simulink library "qss_tb_library_aalto"  (Simulink 8.3)
settings: Solver=ode45  SolverMode=SingleTasking  StartTime=0.0  StopTime=1220  RelTol=1e-3
undefined symbols (not defined in the file): c_BT_E1, c_BT_E2, c_BT_E3, c_BT_E4, c_BT_L1, c_BT_L2, c_BT_L3, c_BT_L4, cap_BT, cc_done, delta_h_C_air, DiscIntNeverNeededParam, dw_GG_c, eff_FC_max, eta_EG_map, eta_EM_map, g, h, H_o_m, H_u, I_BT_max, i_FC_in, i_FC_max, k1, k2, k3, k4, k_cs, M_air, manual_gearbox, P_CVT_opt, power_max, Q_BT_0, Q_BT_IC, Q_BT_min, Q_SC_IC, r_wheel, rchg_map_BT, rdis_map_BT, rho, rho_f, soc_map_BT, t_c, T_CE_max, T_EG_c, T_EG_max, T_EM_max, T_z, U_BT_0, V, V_CE_map, V_FC_out, voc_map_BT, w_CE_max, w_CE_upper, w_CVT_opt, w_EG_row, w_EG_upper, w_EM_row, w_EM_upper ... (+1)
libraries: simulink x4
(part 4 of 4)

== system qss_tb_library_aalto/Vehicle/Vehicle/Rolling resistance ==
  v : Inport
  Rolling resistance : Constant  Value=m_f*g*mu
  Switch : Switch  Criteria=u2 > Threshold  Threshold=eps
  To Workspace2 : ToWorkspace  VariableName=F_roll  SampleTime=-1
  standstill : Constant  Value=0
  F_roll : Outport
  wires:
  Switch/1 -> To Workspace2/1, F_roll/1
  v/1 -> Switch/2
  standstill/1 -> Switch/3
  Rolling resistance/1 -> Switch/1

== system qss_tb_library_aalto/Vehicle/Vehicle v2/Aerodynamic resistance ==
  v : Inport
  Aerodynamic resistance : Fcn  Expr=0.5*rho*cw*A_f*u^2
  To Workspace10 : ToWorkspace  VariableName=F_aero  SampleTime=-1
  F_aero : Outport  InitialOutput=0
  wires:
  Aerodynamic resistance/1 -> To Workspace10/1, F_aero/1
  v/1 -> Aerodynamic resistance/1

== system qss_tb_library_aalto/Vehicle/Vehicle v2/Average speed ==
  v : Inport
  Gain5 : Gain  Gain=0.5  SaturateOnIntegerOverflow=on  OutDataTypeStr=Inherit: Same as input  ParamDataTypeStr=Inherit: Same as input
  Sum2 : Sum  SaturateOnIntegerOverflow=on  InputSameDT=on  OutDataTypeStr=Inherit: Same as first input
  Unit Delay : UnitDelay  SampleTime=h
  v_a : Outport  InitialOutput=0
  wires:
  v/1 -> Unit Delay/1, Sum2/1
  Gain5/1 -> v_a/1
  Sum2/1 -> Gain5/1
  Unit Delay/1 -> Sum2/2

== system qss_tb_library_aalto/Vehicle/Vehicle v2/Inertia ==
  d_v : Inport
  Inertia : Fcn  Expr=m_f*(1+mt2m_f)*u/h
  To Workspace10 : ToWorkspace  VariableName=F_iner  SampleTime=-1
  F_iner : Outport  InitialOutput=0
  wires:
  d_v/1 -> Inertia/1
  Inertia/1 -> To Workspace10/1, F_iner/1

== system qss_tb_library_aalto/Vehicle/Vehicle v2/Rolling resistance ==
  v : Inport
  Rolling resistance : Constant  Value=m_f*g*mu
  Switch : Switch  Criteria=u2 > Threshold  Threshold=eps
  To Workspace2 : ToWorkspace  VariableName=F_roll  SampleTime=-1
  standstill : Constant  Value=0
  F_roll : Outport
  wires:
  Rolling resistance/1 -> Switch/1
  standstill/1 -> Switch/3
  v/1 -> Switch/2
  Switch/1 -> F_roll/1, To Workspace2/1

== system qss_tb_library_aalto/Controller/Battery Controller/Geno-Group On/Clock ==
  Constant : Constant
  Sum : Sum  Inputs=+-  SaturateOnIntegerOverflow=on  InputSameDT=on  OutDataTypeStr=Inherit: Same as first input
  Unit Delay : UnitDelay  SampleTime=duration
  out_1 : Outport  InitialOutput=0
  wires:
  Constant/1 -> Sum/1
  Sum/1 -> Unit Delay/1, out_1/1
  Unit Delay/1 -> Sum/2

== system qss_tb_library_aalto/Controller/Gen-set Controller v2/Engine start control/Engine on off ==
  S : Inport
  R : Inport  Port=2
  Demux : Demux  Outputs=2
  Logic : CombinatorialLogic  TruthTable=[0 1;0 1;1 0;0 1;1 0;0 1;1 0;1 0]
  Memory : Memory  InheritSampleTime=on
  Mux : Mux  Inputs=3
  Q : Outport  InitialOutput=0
  !Q : Outport  Port=2  InitialOutput=1
  wires:
  Mux/1 -> Logic/1
  Logic/1 -> Demux/1
  Demux/2 -> !Q/1
  Demux/1 -> Q/1, Memory/1
  Memory/1 -> Mux/1
  S/1 -> Mux/2
  R/1 -> Mux/3

== system qss_tb_library_aalto/Controller/Gen-set Controller v2/Engine start control/tempo ==
  flag : Inport
  time : Inport  Port=2
  S-R Flip-Flop : Subsystem  mask(SRFlipFlop){initial_condition=1}
      mask prompts: initial_condition "Initial condition (state of Q):"
      mask help: S-R Flip-Flop Block
      mask Help: web([docroot '/toolbox/simulink/ref_extras/srflipflop.html'])
  Terminator : Terminator
  Unit Delay : UnitDelay  SampleTime=h
  __Logical Operator2 : Logic
  __Logical Operator3 : Logic  Operator=NOT
  __Terminator : Terminator
  counter : DiscreteIntegrator  ExternalReset=rising  SampleTime=h  ICPrevOutput=DiscIntNeverNeededParam  ICPrevScaledInput=DiscIntNeverNeededParam
  end of tempo : RelationalOperator  InputSameDT=on
  tempo ok --> 1 : Subsystem  mask(SRFlipFlop){initial_condition=0, Tech=h}
      mask prompts: initial_condition "Initial condition:"; Tech "pas d'echantillonage"
      mask help: S-R Flip Flop Block
  tempo : Outport
  wires:
  S-R Flip-Flop/1(Q) -> counter/1
  flag/1 -> __Logical Operator2/1, tempo ok --> 1/1(S)
  S-R Flip-Flop/2(!Q) -> __Terminator/1
  __Logical Operator2/1 -> S-R Flip-Flop/1(S)
  __Logical Operator3/1 -> __Logical Operator2/2
  time/1 -> end of tempo/2
  end of tempo/1 -> Unit Delay/1, tempo ok --> 1/2(R)
  Unit Delay/1 -> __Logical Operator3/1, S-R Flip-Flop/2(R), counter/2
  counter/1 -> end of tempo/1
  tempo ok --> 1/2(!Q) -> Terminator/1
  tempo ok --> 1/1(Q) -> tempo/1

== system qss_tb_library_aalto/Controller/Gen-set Controller/Engine start control/Engine on off ==
  S : Inport
  R : Inport  Port=2
  Demux : Demux  Outputs=2
  Logic : CombinatorialLogic  TruthTable=[0 1;0 1;1 0;0 1;1 0;0 1;1 0;1 0]
  Memory : Memory  InheritSampleTime=on
  Mux : Mux  Inputs=3
  Q : Outport  InitialOutput=0
  !Q : Outport  Port=2  InitialOutput=1
  wires:
  R/1 -> Mux/3
  S/1 -> Mux/2
  Memory/1 -> Mux/1
  Demux/1 -> Memory/1, Q/1
  Demux/2 -> !Q/1
  Logic/1 -> Demux/1
  Mux/1 -> Logic/1

== system qss_tb_library_aalto/Controller/Gen-set Controller/Engine start control/tempo ==
  flag : Inport
  time : Inport  Port=2
  S-R Flip-Flop : Subsystem  mask(SRFlipFlop){initial_condition=1}
      mask prompts: initial_condition "Initial condition (state of Q):"
      mask help: S-R Flip-Flop Block
      mask Help: web([docroot '/toolbox/simulink/ref_extras/srflipflop.html'])
  Terminator : Terminator
  Unit Delay : UnitDelay  SampleTime=h
  __Logical Operator2 : Logic
  __Logical Operator3 : Logic  Operator=NOT
  __Terminator : Terminator
  counter : DiscreteIntegrator  ExternalReset=rising  SampleTime=h  ICPrevOutput=DiscIntNeverNeededParam  ICPrevScaledInput=DiscIntNeverNeededParam
  end of tempo : RelationalOperator  InputSameDT=on
  tempo ok --> 1 : Subsystem  mask(SRFlipFlop){initial_condition=0, Tech=h}
      mask prompts: initial_condition "Initial condition:"; Tech "pas d'echantillonage"
      mask help: S-R Flip Flop Block
  tempo : Outport
  wires:
  tempo ok --> 1/1(Q) -> tempo/1
  tempo ok --> 1/2(!Q) -> Terminator/1
  counter/1 -> end of tempo/1
  Unit Delay/1 -> counter/2, S-R Flip-Flop/2(R), __Logical Operator3/1
  end of tempo/1 -> tempo ok --> 1/2(R), Unit Delay/1
  time/1 -> end of tempo/2
  __Logical Operator3/1 -> __Logical Operator2/2
  __Logical Operator2/1 -> S-R Flip-Flop/1(S)
  S-R Flip-Flop/2(!Q) -> __Terminator/1
  flag/1 -> tempo ok --> 1/1(S), __Logical Operator2/1
  S-R Flip-Flop/1(Q) -> counter/1

== system qss_tb_library_aalto/Energy Buffer/Battery/Battery voltage/Charging ==
  Q_BT : Inport
  P_BT : Inport  Port=2
  Enable : EnablePort
  Constant4 : Constant  Value=Q_BT_0
  Fcn : Fcn  Expr=(c_BT_L3*u[1]+c_BT_L1+sqrt((c_BT_L3*u[1]+c_BT_L1)^2+4*(c_BT_L4*u[1]+c_BT_L2)*(-u[2])))/2
  Gain2 : Gain  Gain=1/Q_BT_0  SaturateOnIntegerOverflow=on  OutDataTypeStr=Inherit: Same as input  ParamDataTypeStr=Inherit: Same as input
  Gain4 : Gain  Gain=1/I_0  SaturateOnIntegerOverflow=on  OutDataTypeStr=Inherit: Same as input  ParamDataTypeStr=Inherit: Same as input
  Mux : Mux  Inputs=2
  Sum4 : Sum  Inputs=-+  SaturateOnIntegerOverflow=on  InputSameDT=on  OutDataTypeStr=Inherit: Same as first input
  U_BT_L : Outport  InitialOutput=0
  wires:
  Gain4/1 -> Mux/2
  Gain2/1 -> Mux/1
  Sum4/1 -> Gain2/1
  Q_BT/1 -> Sum4/1
  Constant4/1 -> Sum4/2
  P_BT/1 -> Gain4/1
  Mux/1 -> Fcn/1
  Fcn/1 -> U_BT_L/1

== system qss_tb_library_aalto/Energy Buffer/Battery/Battery voltage/Discharging ==
  note: q
  note: P/I_0
  Q_BT : Inport
  P_BT : Inport  Port=2
  Enable : EnablePort
  Constant6 : Constant  Value=Q_BT_0
  Fcn : Fcn  Expr=(c_BT_E3*u[1]+c_BT_E1+sqrt((c_BT_E3*u[1]+c_BT_E1)^2+4*(c_BT_E4*u[1]+c_BT_E2)*(-u[2])))/2
  Gain4 : Gain  Gain=1/Q_BT_0  SaturateOnIntegerOverflow=on  OutDataTypeStr=Inherit: Same as input  ParamDataTypeStr=Inherit: Same as input
  Gain5 : Gain  Gain=1/I_0  SaturateOnIntegerOverflow=on  OutDataTypeStr=Inherit: Same as input  ParamDataTypeStr=Inherit: Same as input
  Mux : Mux  Inputs=2
  Sum7 : Sum  Inputs=-+  SaturateOnIntegerOverflow=on  InputSameDT=on  OutDataTypeStr=Inherit: Same as first input
  U_BT_E : Outport  InitialOutput=0
  wires:
  Fcn/1 -> U_BT_E/1
  Sum7/1 -> Gain4/1
  Q_BT/1 -> Sum7/1
  Constant6/1 -> Sum7/2
  P_BT/1 -> Gain5/1
  Gain4/1 -> Mux/1
  Gain5/1 -> Mux/2
  Mux/1 -> Fcn/1

== system qss_tb_library_aalto/Energy Buffer/Battery/Battery voltage/Enable charging ==
  P_BT : Inport
  Gain : Gain  Gain=-1  SaturateOnIntegerOverflow=on  OutDataTypeStr=Inherit: Same as input  ParamDataTypeStr=Inherit: Same as input
  Saturation : Saturate  UpperLimit=0  LowerLimit=-inf
  Sign : Signum
  e_E : Outport  InitialOutput=0
  wires:
  P_BT/1 -> Saturation/1
  Sign/1 -> e_E/1
  Saturation/1 -> Gain/1
  Gain/1 -> Sign/1

== system qss_tb_library_aalto/Energy Buffer/Battery/Battery voltage/Enable discharging ==
  P_BT : Inport
  Saturation : Saturate  UpperLimit=inf  LowerLimit=0
  Sign : Signum
  e_E : Outport  InitialOutput=0
  wires:
  P_BT/1 -> Saturation/1
  Sign/1 -> e_E/1
  Saturation/1 -> Sign/1

== system qss_tb_library_aalto/Energy Buffer/Battery/Battery voltage/Enable idle ==
  P_BT : Inport
  Abs : Abs  SaturateOnIntegerOverflow=on
  Constant : Constant
  Sign : Signum
  Sum4 : Sum  Inputs=-+  SaturateOnIntegerOverflow=on  InputSameDT=on  OutDataTypeStr=Inherit: Same as first input
  e_Z : Outport  InitialOutput=0
  wires:
  P_BT/1 -> Sign/1
  Sign/1 -> Abs/1
  Abs/1 -> Sum4/1
  Sum4/1 -> e_Z/1
  Constant/1 -> Sum4/2

== system qss_tb_library_aalto/Energy Buffer/Battery/Battery voltage/Idle ==
  Q_BT : Inport
  Enable : EnablePort  StatesWhenEnabling=reset
  Constant : Constant  Value=c_BT_L1
  Constant6 : Constant  Value=Q_BT_0
  Gain4 : Gain  Gain=c_BT_L3/Q_BT_0  SaturateOnIntegerOverflow=on  OutDataTypeStr=Inherit: Same as input  ParamDataTypeStr=Inherit: Same as input
  Sum7 : Sum  Inputs=-+  SaturateOnIntegerOverflow=on  InputSameDT=on  OutDataTypeStr=Inherit: Same as first input
  Sum8 : Sum  SaturateOnIntegerOverflow=on  InputSameDT=on  OutDataTypeStr=Inherit: Same as first input
  U_BT_E : Outport  InitialOutput=0
  wires:
  Sum7/1 -> Gain4/1
  Q_BT/1 -> Sum7/1
  Constant6/1 -> Sum7/2
  Gain4/1 -> Sum8/1
  Constant/1 -> Sum8/2
  Sum8/1 -> U_BT_E/1

== system qss_tb_library_aalto/Energy Buffer/Battery/Battery voltage/Supervision battery ==
  Q_BT : Inport
  U_BT : Inport  Port=2
  I_BT : Inport  Port=3
  Abs : Abs  SaturateOnIntegerOverflow=on
  Constant4 : Constant  Value=Q_BT_0
  Constant6 : Constant  Value=c_BT_E1
  Constant7 : Constant  Value=I_BT_max
  Gain2 : Gain  Gain=c_BT_E3/Q_BT_0  SaturateOnIntegerOverflow=on  OutDataTypeStr=Inherit: Same as input  ParamDataTypeStr=Inherit: Same as input
  Gain3 : Gain  Gain=2  SaturateOnIntegerOverflow=on  OutDataTypeStr=Inherit: Same as input  ParamDataTypeStr=Inherit: Same as input
  Saturation : Saturate  UpperLimit=0  LowerLimit=-inf
  Saturation1 : Saturate  UpperLimit=0  LowerLimit=-inf
  Stop Simulation : Stop
  Stop Simulation1 : Stop
  Sum1 : Sum  Inputs=-+  SaturateOnIntegerOverflow=on  InputSameDT=on  OutDataTypeStr=Inherit: Same as first input
  Sum2 : Sum  Inputs=+-  SaturateOnIntegerOverflow=on  InputSameDT=on  OutDataTypeStr=Inherit: Same as first input
  Sum3 : Sum  SaturateOnIntegerOverflow=on  InputSameDT=on  OutDataTypeStr=Inherit: Same as first input
  Sum4 : Sum  Inputs=-+  SaturateOnIntegerOverflow=on  InputSameDT=on  OutDataTypeStr=Inherit: Same as first input
  wires:
  Sum3/1 -> Sum1/1
  U_BT/1 -> Gain3/1
  Gain3/1 -> Sum1/2
  Saturation/1 -> Stop Simulation1/1
  Saturation1/1 -> Stop Simulation/1
  Sum1/1 -> Saturation1/1
  Constant6/1 -> Sum3/2
  Gain2/1 -> Sum3/1
  Sum4/1 -> Gain2/1
  Q_BT/1 -> Sum4/1
  Constant4/1 -> Sum4/2
  Constant7/1 -> Sum2/1
  Sum2/1 -> Saturation/1
  I_BT/1 -> Abs/1
  Abs/1 -> Sum2/2

== system qss_tb_library_aalto/Energy Buffer/Battery v2/cell model/soc calculation ==
  current : Inport
  (sec->hrs) : Gain  Gain=1/3600  SaturateOnIntegerOverflow=on  OutDataTypeStr=Inherit: Same as input  ParamDataTypeStr=Inherit: Same as input
  (sec->hrs)1 : Gain  Gain=-1  SaturateOnIntegerOverflow=on  OutDataTypeStr=Inherit: Same as input  ParamDataTypeStr=Inherit: Same as input
  0 <= SOC <= 1 : Saturate  UpperLimit=1  LowerLimit=0
  Constant : Constant  Value=init_soc_BT
  Constant1 : Constant  Value=cap_BT
  Discrete-Time Integrator : DiscreteIntegrator  InitialConditionSource=external  ICPrevOutput=DiscIntNeverNeededParam  ICPrevScaledInput=DiscIntNeverNeededParam
  Divide : Product  Inputs=*/  RndMeth=Zero
  Product : Product  RndMeth=Zero
  soc : Outport
  wires:
  current/1 -> (sec->hrs)/1
  0 <= SOC <= 1/1 -> soc/1
  (sec->hrs)/1 -> (sec->hrs)1/1
  Discrete-Time Integrator/1 -> Divide/1
  Divide/1 -> 0 <= SOC <= 1/1
  Constant/1 -> Product/1
  Product/1 -> Discrete-Time Integrator/2
  (sec->hrs)1/1 -> Discrete-Time Integrator/1
  Constant1/1 -> Product/2, Divide/2

== system qss_tb_library_aalto/Energy Buffer/Battery v2/cell model/voltage calculation ==
  note: Volt = Voc - Rint*I
  SOC (prev) : Inport
  Current : Inport  Port=2
  Product2 : Product  SaturateOnIntegerOverflow=on  InputSameDT=on  OutDataTypeStr=Inherit: Same as first input
  Rchg : Lookup  InputValues=soc_map_BT  Table=rchg_map_BT  SaturateOnIntegerOverflow=on
  Rdis : Lookup  InputValues=soc_map_BT  Table=rdis_map_BT  SaturateOnIntegerOverflow=on
  Sum1 : Sum  Inputs=+-  SaturateOnIntegerOverflow=on  InputSameDT=on  OutDataTypeStr=Inherit: Same as first input
  Switch : Switch  SaturateOnIntegerOverflow=on  InputSameDT=on
  Switch1 : Switch  SaturateOnIntegerOverflow=on  InputSameDT=on
  VOC : Lookup  InputValues=soc_map_BT  Table=voc_map_BT  SaturateOnIntegerOverflow=on
  coulombic efficiency : Gain  Gain=0.99
  Voc : Outport  InitialOutput=0
  voltage : Outport  Port=2  InitialOutput=0
  Rint : Outport  Port=3  InitialOutput=0
  wires:
  Switch/1 -> Rint/1, Product2/2
  Rdis/1 -> Switch/1
  Rchg/1 -> Switch/3
  VOC/1 -> Voc/1, Sum1/1
  SOC (prev)/1 -> VOC/1, Rdis/1, Rchg/1
  Product2/1 -> Sum1/2
  Sum1/1 -> voltage/1
  Switch1/1 -> Switch/2, Product2/1
  Current/1 -> Switch1/2, Switch1/1, coulombic efficiency/1
  coulombic efficiency/1 -> Switch1/3

== system qss_tb_library_aalto/Energy Buffer/Battery v3/cell model/soc calculation ==
  current : Inport
  (sec->hrs) : Gain  Gain=1/3600  SaturateOnIntegerOverflow=on  OutDataTypeStr=Inherit: Same as input  ParamDataTypeStr=Inherit: Same as input
  (sec->hrs)1 : Gain  Gain=-1  SaturateOnIntegerOverflow=on  OutDataTypeStr=Inherit: Same as input  ParamDataTypeStr=Inherit: Same as input
  0 <= SOC <= 1 : Saturate  UpperLimit=1  LowerLimit=0
  Constant : Constant  Value=init_soc_BT
  Constant1 : Constant  Value=cap_BT
  Discrete-Time Integrator : DiscreteIntegrator  InitialConditionSource=external  ICPrevOutput=DiscIntNeverNeededParam  ICPrevScaledInput=DiscIntNeverNeededParam
  Divide : Product  Inputs=*/  RndMeth=Zero
  Product : Product  RndMeth=Zero
  soc : Outport
  wires:
  Constant1/1 -> Divide/2, Product/2
  (sec->hrs)1/1 -> Discrete-Time Integrator/1
  Product/1 -> Discrete-Time Integrator/2
  Constant/1 -> Product/1
  Divide/1 -> 0 <= SOC <= 1/1
  Discrete-Time Integrator/1 -> Divide/1
  (sec->hrs)/1 -> (sec->hrs)1/1
  0 <= SOC <= 1/1 -> soc/1
  current/1 -> (sec->hrs)/1

== system qss_tb_library_aalto/Energy Buffer/Battery v3/cell model/voltage calculation ==
  note: Volt = Voc - Rint*I
  SOC (prev) : Inport
  Current : Inport  Port=2
  Product2 : Product  SaturateOnIntegerOverflow=on  InputSameDT=on  OutDataTypeStr=Inherit: Same as first input
  Rchg : Lookup  InputValues=soc_map_BT  Table=rchg_map_BT  SaturateOnIntegerOverflow=on
  Rdis : Lookup  InputValues=soc_map_BT  Table=rdis_map_BT  SaturateOnIntegerOverflow=on
  Sum1 : Sum  Inputs=+-  SaturateOnIntegerOverflow=on  InputSameDT=on  OutDataTypeStr=Inherit: Same as first input
  Switch : Switch  SaturateOnIntegerOverflow=on  InputSameDT=on
  VOC : Lookup  InputValues=soc_map_BT  Table=voc_map_BT  SaturateOnIntegerOverflow=on
  Voc : Outport  InitialOutput=0
  voltage : Outport  Port=2  InitialOutput=0
  Rint : Outport  Port=3  InitialOutput=0
  wires:
  Current/1 -> Product2/1, Switch/2
  Sum1/1 -> voltage/1
  Product2/1 -> Sum1/2
  SOC (prev)/1 -> Rchg/1, Rdis/1, VOC/1
  VOC/1 -> Sum1/1, Voc/1
  Rchg/1 -> Switch/3
  Rdis/1 -> Switch/1
  Switch/1 -> Product2/2, Rint/1

== system qss_tb_library_aalto/Energy Converter/Combustion Engine (hybrid vehicle)/torque limit/saturation with inputs ==
  upper limit in : Inport
  signal in : Inport  Port=2
  lower limit in : Inport  Port=3
  Relational Operator : RelationalOperator  Operator=<  InputSameDT=on
  Relational Operator1 : RelationalOperator  InputSameDT=on
  Switch : Switch  Threshold=0.5  SaturateOnIntegerOverflow=on  InputSameDT=on
  Switch1 : Switch  Threshold=0.5  SaturateOnIntegerOverflow=on  InputSameDT=on
  signal out : Outport
  wires:
  Switch/1 -> Switch1/1, Relational Operator1/1
  signal in/1 -> Switch/3, Relational Operator/2
  Switch1/1 -> signal out/1
  Relational Operator1/1 -> Switch1/2
  Relational Operator/1 -> Switch/2
  lower limit in/1 -> Switch1/3, Relational Operator1/2
  upper limit in/1 -> Switch/1, Relational Operator/1

== system qss_tb_library_aalto/Energy Converter/Combustion Engine (hybrid vehicle) v2/torque limit/saturation with inputs ==
  upper limit in : Inport
  signal in : Inport  Port=2
  lower limit in : Inport  Port=3
  Relational Operator : RelationalOperator  Operator=<  InputSameDT=on
  Relational Operator1 : RelationalOperator  InputSameDT=on
  Switch : Switch  Threshold=0.5  SaturateOnIntegerOverflow=on  InputSameDT=on
  Switch1 : Switch  Threshold=0.5  SaturateOnIntegerOverflow=on  InputSameDT=on
  signal out : Outport
  wires:
  upper limit in/1 -> Relational Operator/1, Switch/1
  lower limit in/1 -> Relational Operator1/2, Switch1/3
  Relational Operator/1 -> Switch/2
  Relational Operator1/1 -> Switch1/2
  Switch1/1 -> signal out/1
  signal in/1 -> Relational Operator/2, Switch/3
  Switch/1 -> Relational Operator1/1, Switch1/1

== system qss_tb_library_aalto/Gear System/Continuously Variable Transmission/Power flow/Engine -> Wheel ==
  w_wheel : Inport
  T_wheel : Inport  Port=2
  j_CVT : Inport  Port=3
  Constant3 : Constant  Value=P_CVT0
  Constant4 : Constant  Value=inf
  Gain : Gain  Gain=e_CVT  SaturateOnIntegerOverflow=on  OutDataTypeStr=Inherit: Same as input  ParamDataTypeStr=Inherit: Same as input
  Product4 : Product  Inputs=*/  SaturateOnIntegerOverflow=on  RndMeth=Zero  InputSameDT=on  OutDataTypeStr=Inherit: Same as first input
  Product5 : Product  Inputs=/*  SaturateOnIntegerOverflow=on  RndMeth=Zero  InputSameDT=on  OutDataTypeStr=Inherit: Same as first input
  Sum1 : Sum  SaturateOnIntegerOverflow=on  InputSameDT=on  OutDataTypeStr=Inherit: Same as first input
  Switch2 : Switch  Threshold=w_wheel_min  SaturateOnIntegerOverflow=on  InputSameDT=on
  T_CVT+ : Outport  InitialOutput=0
  wires:
  Gain/1 -> Product4/2
  Product4/1 -> T_CVT+/1
  Sum1/1 -> Product4/1
  T_wheel/1 -> Sum1/2
  Product5/1 -> Sum1/1
  w_wheel/1 -> Switch2/1, Switch2/2
  Constant4/1 -> Switch2/3
  Switch2/1 -> Product5/1
  Constant3/1 -> Product5/2
  j_CVT/1 -> Gain/1

== system qss_tb_library_aalto/Gear System/Continuously Variable Transmission/Power flow/Pwer Wheel -> Engine ==
  w_wheel : Inport
  T_wheel : Inport  Port=2
  j_CVT : Inport  Port=3
  Constant1 : Constant  Value=P_CVT0
  Constant2 : Constant  Value=inf
  Gain1 : Gain  Gain=1/e_CVT  SaturateOnIntegerOverflow=on  OutDataTypeStr=Inherit: Same as input  ParamDataTypeStr=Inherit: Same as input
  Gain2 : Gain  Gain=1/e_CVT  SaturateOnIntegerOverflow=on  OutDataTypeStr=Inherit: Same as input  ParamDataTypeStr=Inherit: Same as input
  Product2 : Product  Inputs=*/  SaturateOnIntegerOverflow=on  RndMeth=Zero  InputSameDT=on  OutDataTypeStr=Inherit: Same as first input
  Product3 : Product  Inputs=/*  SaturateOnIntegerOverflow=on  RndMeth=Zero  InputSameDT=on  OutDataTypeStr=Inherit: Same as first input
  Sum : Sum  Inputs=-+  SaturateOnIntegerOverflow=on  InputSameDT=on  OutDataTypeStr=Inherit: Same as first input
  Switch1 : Switch  Threshold=w_wheel_min  SaturateOnIntegerOverflow=on  InputSameDT=on
  T_CVT- : Outport  InitialOutput=0
  wires:
  Sum/1 -> Product2/1
  Gain1/1 -> Product3/2
  Switch1/1 -> Product3/1
  T_wheel/1 -> Sum/2
  Product3/1 -> Sum/1
  Product2/1 -> T_CVT-/1
  w_wheel/1 -> Switch1/1, Switch1/2
  Constant1/1 -> Gain1/1
  Constant2/1 -> Switch1/3
  j_CVT/1 -> Gain2/1
  Gain2/1 -> Product2/2

== system qss_tb_library_aalto/Gear System/Manual Gear Box/Power flow/Engine -> Wheel ==
  w_wheel : Inport
  T_wheel : Inport  Port=2
  gear : Inport  Port=3
  Constant1 : Constant  Value=P_GT0
  Constant2 : Constant  Value=inf
  Gain : Gain  Gain=e_GT  SaturateOnIntegerOverflow=on  OutDataTypeStr=Inherit: Same as input  ParamDataTypeStr=Inherit: Same as input
  Product2 : Product  Inputs=*/  SaturateOnIntegerOverflow=on  RndMeth=Zero  InputSameDT=on  OutDataTypeStr=Inherit: Same as first input
  Product3 : Product  Inputs=/*  SaturateOnIntegerOverflow=on  RndMeth=Zero  InputSameDT=on  OutDataTypeStr=Inherit: Same as first input
  Sum : Sum  SaturateOnIntegerOverflow=on  InputSameDT=on  OutDataTypeStr=Inherit: Same as first input
  Switch1 : Switch  Threshold=w_wheel_min  SaturateOnIntegerOverflow=on  InputSameDT=on
  T_MGB+ : Outport  InitialOutput=0
  wires:
  T_wheel/1 -> Sum/2
  Product3/1 -> Sum/1
  Gain/1 -> Product2/2
  Product2/1 -> T_MGB+/1
  Sum/1 -> Product2/1
  w_wheel/1 -> Switch1/2, Switch1/1
  Constant2/1 -> Switch1/3
  Switch1/1 -> Product3/1
  Constant1/1 -> Product3/2
  gear/1 -> Gain/1

== system qss_tb_library_aalto/Gear System/Manual Gear Box/Power flow/Wheel -> Engine ==
  w_wheel : Inport
  T_wheel : Inport  Port=2
  gear : Inport  Port=3
  Constant1 : Constant  Value=P_GT0
  Constant2 : Constant  Value=inf
  Gain1 : Gain  Gain=e_GT  SaturateOnIntegerOverflow=on  OutDataTypeStr=Inherit: Same as input  ParamDataTypeStr=Inherit: Same as input
  Gain2 : Gain  Gain=1/e_GT  SaturateOnIntegerOverflow=on  OutDataTypeStr=Inherit: Same as input  ParamDataTypeStr=Inherit: Same as input
  Product2 : Product  Inputs=*/  SaturateOnIntegerOverflow=on  RndMeth=Zero  InputSameDT=on  OutDataTypeStr=Inherit: Same as first input
  Product3 : Product  Inputs=/*  SaturateOnIntegerOverflow=on  RndMeth=Zero  InputSameDT=on  OutDataTypeStr=Inherit: Same as first input
  Sum : Sum  SaturateOnIntegerOverflow=on  InputSameDT=on  OutDataTypeStr=Inherit: Same as first input
  Switch1 : Switch  Threshold=w_wheel_min  SaturateOnIntegerOverflow=on  InputSameDT=on
  T_MGB- : Outport  InitialOutput=0
  wires:
  w_wheel/1 -> Switch1/1, Switch1/2
  gear/1 -> Gain2/1
  Constant2/1 -> Switch1/3
  Switch1/1 -> Gain1/1
  Constant1/1 -> Product3/2
  T_wheel/1 -> Sum/1
  Gain2/1 -> Product2/2
  Product2/1 -> T_MGB-/1
  Product3/1 -> Sum/2
  Sum/1 -> Product2/1
  Gain1/1 -> Product3/1

== system qss_tb_library_aalto/Gear System/Simple Transmission/Power flow/Energy Engine -> Wheel ==
  w_wheel : Inport
  T_wheel : Inport  Port=2
  gear_ratio : Inport  Port=3
  Constant1 : Constant  Value=P_GT0
  Constant2 : Constant  Value=inf
  Gain : Gain  Gain=e_GT  SaturateOnIntegerOverflow=on  OutDataTypeStr=Inherit: Same as input  ParamDataTypeStr=Inherit: Same as input
  Product2 : Product  Inputs=*/  SaturateOnIntegerOverflow=on  RndMeth=Zero  InputSameDT=on  OutDataTypeStr=Inherit: Same as first input
  Product3 : Product  Inputs=/*  SaturateOnIntegerOverflow=on  RndMeth=Zero  InputSameDT=on  OutDataTypeStr=Inherit: Same as first input
  Sum : Sum  SaturateOnIntegerOverflow=on  InputSameDT=on  OutDataTypeStr=Inherit: Same as first input
  Switch1 : Switch  Threshold=w_wheel_min  SaturateOnIntegerOverflow=on  InputSameDT=on
  T_trans+ : Outport  InitialOutput=0
  wires:
  T_wheel/1 -> Sum/2
  Product3/1 -> Sum/1
  Gain/1 -> Product2/2
  Product2/1 -> T_trans+/1
  Sum/1 -> Product2/1
  w_wheel/1 -> Switch1/2, Switch1/1
  Constant2/1 -> Switch1/3
  Switch1/1 -> Product3/1
  Constant1/1 -> Product3/2
  gear_ratio/1 -> Gain/1

== system qss_tb_library_aalto/Gear System/Simple Transmission/Power flow/Energy Wheel -> Engine ==
  w_wheel : Inport
  T_wheel : Inport  Port=2
  gear_ratio : Inport  Port=3
  Constant1 : Constant  Value=P_GT0
  Constant2 : Constant  Value=inf
  Gain1 : Gain  Gain=e_GT  SaturateOnIntegerOverflow=on  OutDataTypeStr=Inherit: Same as input  ParamDataTypeStr=Inherit: Same as input
  Gain2 : Gain  Gain=1/e_GT  SaturateOnIntegerOverflow=on  OutDataTypeStr=Inherit: Same as input  ParamDataTypeStr=Inherit: Same as input
  Product2 : Product  Inputs=*/  SaturateOnIntegerOverflow=on  RndMeth=Zero  InputSameDT=on  OutDataTypeStr=Inherit: Same as first input
  Product3 : Product  Inputs=/*  SaturateOnIntegerOverflow=on  RndMeth=Zero  InputSameDT=on  OutDataTypeStr=Inherit: Same as first input
  Sum : Sum  SaturateOnIntegerOverflow=on  InputSameDT=on  OutDataTypeStr=Inherit: Same as first input
  Switch1 : Switch  Threshold=w_wheel_min  SaturateOnIntegerOverflow=on  InputSameDT=on
  T_trans- : Outport  InitialOutput=0
  wires:
  w_wheel/1 -> Switch1/1, Switch1/2
  gear_ratio/1 -> Gain2/1
  Constant2/1 -> Switch1/3
  Switch1/1 -> Gain1/1
  Constant1/1 -> Product3/2
  T_wheel/1 -> Sum/1
  Gain2/1 -> Product2/2
  Product2/1 -> T_trans-/1
  Product3/1 -> Sum/2
  Sum/1 -> Product2/1
  Gain1/1 -> Product3/1

== system qss_tb_library_aalto/Gear System/Transmission CE-EG/Power flow/Energy Engine -> Wheel ==
  w_wheel : Inport
  T_wheel : Inport  Port=2
  gear_ratio : Inport  Port=3
  Constant1 : Constant  Value=P_GT0
  Constant2 : Constant  Value=inf
  Gain1 : Gain  Gain=e_GT  SaturateOnIntegerOverflow=on  OutDataTypeStr=Inherit: Same as input  ParamDataTypeStr=Inherit: Same as input
  Lower limit : Saturate  UpperLimit=inf  LowerLimit=0
  Product2 : Product  Inputs=*/  SaturateOnIntegerOverflow=on  RndMeth=Zero  InputSameDT=on  OutDataTypeStr=Inherit: Same as first input
  Product3 : Product  Inputs=/*  SaturateOnIntegerOverflow=on  RndMeth=Zero  InputSameDT=on  OutDataTypeStr=Inherit: Same as first input
  Sum : Sum  Inputs=-+  SaturateOnIntegerOverflow=on  InputSameDT=on  OutDataTypeStr=Inherit: Same as first input
  Switch1 : Switch  Threshold=w_wheel_min+eps  SaturateOnIntegerOverflow=on  InputSameDT=on
  T_trans+ : Outport  InitialOutput=0
  wires:
  gear_ratio/1 -> Product2/2
  Constant1/1 -> Product3/2
  Switch1/1 -> Product3/1
  Constant2/1 -> Switch1/3
  w_wheel/1 -> Switch1/1, Switch1/2
  Sum/1 -> Product2/1
  Product2/1 -> Gain1/1
  T_wheel/1 -> Sum/2
  Gain1/1 -> Lower limit/1
  Product3/1 -> Sum/1
  Lower limit/1 -> T_trans+/1

== system qss_tb_library_aalto/Gear System/Transmission CE-EG/Power flow/Energy Wheel -> Engine ==
  w_wheel : Inport
  T_wheel : Inport  Port=2
  gear_ratio : Inport  Port=3
  Constant1 : Constant  Value=P_GT0
  Constant2 : Constant  Value=inf
  Gain1 : Gain  Gain=1/e_GT  SaturateOnIntegerOverflow=on  OutDataTypeStr=Inherit: Same as input  ParamDataTypeStr=Inherit: Same as input
  Product2 : Product  Inputs=*/  SaturateOnIntegerOverflow=on  RndMeth=Zero  InputSameDT=on  OutDataTypeStr=Inherit: Same as first input
  Product3 : Product  Inputs=/*  SaturateOnIntegerOverflow=on  RndMeth=Zero  InputSameDT=on  OutDataTypeStr=Inherit: Same as first input
  Sum : Sum  SaturateOnIntegerOverflow=on  InputSameDT=on  OutDataTypeStr=Inherit: Same as first input
  Switch1 : Switch  Threshold=w_wheel_min+eps  SaturateOnIntegerOverflow=on  InputSameDT=on
  T_trans- : Outport  InitialOutput=0
  wires:
  Sum/1 -> Product2/1
  Product3/1 -> Sum/2
  Product2/1 -> Gain1/1
  T_wheel/1 -> Sum/1
  Constant1/1 -> Product3/2
  Switch1/1 -> Product3/1
  Constant2/1 -> Switch1/3
  gear_ratio/1 -> Product2/2
  w_wheel/1 -> Switch1/2, Switch1/1
  Gain1/1 -> T_trans-/1

== system qss_tb_library_aalto/Gear System/Transmission CE-EG v2/Power flow/Energy Engine -> Generator ==
  w_wheel : Inport
  T_wheel : Inport  Port=2
  gear_ratio : Inport  Port=3
  Constant1 : Constant  Value=P_GT0
  Constant2 : Constant  Value=inf
  Gain1 : Gain  Gain=e_GT  SaturateOnIntegerOverflow=on  OutDataTypeStr=Inherit: Same as input  ParamDataTypeStr=Inherit: Same as input
  Product2 : Product  Inputs=*/  SaturateOnIntegerOverflow=on  RndMeth=Zero  InputSameDT=on  OutDataTypeStr=Inherit: Same as first input
  Product3 : Product  Inputs=/*  SaturateOnIntegerOverflow=on  RndMeth=Zero  InputSameDT=on  OutDataTypeStr=Inherit: Same as first input
  Sum : Sum  Inputs=-+  SaturateOnIntegerOverflow=on  InputSameDT=on  OutDataTypeStr=Inherit: Same as first input
  Switch1 : Switch  Threshold=w_wheel_min+eps  SaturateOnIntegerOverflow=on  InputSameDT=on
  T_trans+ : Outport  InitialOutput=0
  wires:
  Gain1/1 -> T_trans+/1
  Product3/1 -> Sum/1
  T_wheel/1 -> Sum/2
  Product2/1 -> Gain1/1
  Sum/1 -> Product2/1
  w_wheel/1 -> Switch1/2, Switch1/1
  Constant2/1 -> Switch1/3
  Switch1/1 -> Product3/1
  Constant1/1 -> Product3/2
  gear_ratio/1 -> Product2/2

== system qss_tb_library_aalto/Gear System/Transmission CE-EG v2/Power flow/Energy Generator -> Engine ==
  w_wheel : Inport
  T_wheel : Inport  Port=2
  gear_ratio : Inport  Port=3
  Constant1 : Constant  Value=P_GT0
  Constant2 : Constant  Value=inf
  Gain1 : Gain  Gain=1/e_GT  SaturateOnIntegerOverflow=on  OutDataTypeStr=Inherit: Same as input  ParamDataTypeStr=Inherit: Same as input
  Product2 : Product  Inputs=*/  SaturateOnIntegerOverflow=on  RndMeth=Zero  InputSameDT=on  OutDataTypeStr=Inherit: Same as first input
  Product3 : Product  Inputs=/*  SaturateOnIntegerOverflow=on  RndMeth=Zero  InputSameDT=on  OutDataTypeStr=Inherit: Same as first input
  Sum : Sum  SaturateOnIntegerOverflow=on  InputSameDT=on  OutDataTypeStr=Inherit: Same as first input
  Switch1 : Switch  Threshold=w_wheel_min+eps  SaturateOnIntegerOverflow=on  InputSameDT=on
  T_trans- : Outport  InitialOutput=0
  wires:
  Gain1/1 -> T_trans-/1
  w_wheel/1 -> Switch1/1, Switch1/2
  gear_ratio/1 -> Product2/2
  Constant2/1 -> Switch1/3
  Switch1/1 -> Product3/1
  Constant1/1 -> Product3/2
  T_wheel/1 -> Sum/1
  Product2/1 -> Gain1/1
  Product3/1 -> Sum/2
  Sum/1 -> Product2/1

== system qss_tb_library_aalto/Gear System/Transmission Vehicle-EM/Power flow/Energy Engine -> Wheel ==
  w_wheel : Inport
  T_wheel : Inport  Port=2
  gear_ratio : Inport  Port=3
  Constant1 : Constant  Value=P_GT0
  Constant2 : Constant  Value=inf
  Gain : Gain  Gain=e_GT  SaturateOnIntegerOverflow=on  OutDataTypeStr=Inherit: Same as input  ParamDataTypeStr=Inherit: Same as input
  Product2 : Product  Inputs=*/  SaturateOnIntegerOverflow=on  RndMeth=Zero  InputSameDT=on  OutDataTypeStr=Inherit: Same as first input
  Product3 : Product  Inputs=/*  SaturateOnIntegerOverflow=on  RndMeth=Zero  InputSameDT=on  OutDataTypeStr=Inherit: Same as first input
  Sum : Sum  SaturateOnIntegerOverflow=on  InputSameDT=on  OutDataTypeStr=Inherit: Same as first input
  Switch1 : Switch  Threshold=w_wheel_min  SaturateOnIntegerOverflow=on  InputSameDT=on
  T_trans+ : Outport  InitialOutput=0
  wires:
  gear_ratio/1 -> Gain/1
  Constant1/1 -> Product3/2
  Switch1/1 -> Product3/1
  Constant2/1 -> Switch1/3
  w_wheel/1 -> Switch1/1, Switch1/2
  Sum/1 -> Product2/1
  Product2/1 -> T_trans+/1
  Gain/1 -> Product2/2
  Product3/1 -> Sum/1
  T_wheel/1 -> Sum/2

== system qss_tb_library_aalto/Gear System/Transmission Vehicle-EM/Power flow/Energy Wheel -> Engine ==
  w_wheel : Inport
  T_wheel : Inport  Port=2
  gear_ratio : Inport  Port=3
  Constant1 : Constant  Value=P_GT0
  Constant2 : Constant  Value=inf
  Gain1 : Gain  Gain=e_GT  SaturateOnIntegerOverflow=on  OutDataTypeStr=Inherit: Same as input  ParamDataTypeStr=Inherit: Same as input
  Gain2 : Gain  Gain=1/e_GT  SaturateOnIntegerOverflow=on  OutDataTypeStr=Inherit: Same as input  ParamDataTypeStr=Inherit: Same as input
  Product2 : Product  Inputs=*/  SaturateOnIntegerOverflow=on  RndMeth=Zero  InputSameDT=on  OutDataTypeStr=Inherit: Same as first input
  Product3 : Product  Inputs=/*  SaturateOnIntegerOverflow=on  RndMeth=Zero  InputSameDT=on  OutDataTypeStr=Inherit: Same as first input
  Sum : Sum  SaturateOnIntegerOverflow=on  InputSameDT=on  OutDataTypeStr=Inherit: Same as first input
  Switch1 : Switch  Threshold=w_wheel_min  SaturateOnIntegerOverflow=on  InputSameDT=on
  T_trans- : Outport  InitialOutput=0
  wires:
  Gain1/1 -> Product3/1
  Sum/1 -> Product2/1
  Product3/1 -> Sum/2
  Product2/1 -> T_trans-/1
  Gain2/1 -> Product2/2
  T_wheel/1 -> Sum/1
  Constant1/1 -> Product3/2
  Switch1/1 -> Gain1/1
  Constant2/1 -> Switch1/3
  gear_ratio/1 -> Gain2/1
  w_wheel/1 -> Switch1/2, Switch1/1

== system qss_tb_library_aalto/Controller/Gen-set Controller v2/Engine start control/tempo/S-R Flip-Flop ==
  S : Inport
  R : Inport  Port=2
  Demux2 : Demux  Outputs=2
  Logic : CombinatorialLogic  TruthTable=[0 1;1 0;0 1;0 1;1 0;1 0;0 0;0 0]
  Mux2 : Mux  Inputs=3
  Unit Delay : UnitDelay  InitialCondition=initial_condition  SampleTime=-1
  Q : Outport  InitialOutput=0
  !Q : Outport  Port=2  InitialOutput=1
  wires:
  Unit Delay/1 -> Mux2/3
  Mux2/1 -> Logic/1
  Logic/1 -> Demux2/1
  Demux2/2 -> !Q/1
  Demux2/1 -> Q/1, Unit Delay/1
  S/1 -> Mux2/1
  R/1 -> Mux2/2

== system qss_tb_library_aalto/Controller/Gen-set Controller v2/Engine start control/tempo/tempo ok --> 1 ==
  S : Inport
  R : Inport  Port=2
  Demux2 : Demux  Outputs=2
  Logic : CombinatorialLogic  TruthTable=[0 1;0 1;1 0;0 1;1 0;0 1;1 0;1 0]
  Mux2 : Mux  Inputs=3
  Unit Delay1 : UnitDelay  InitialCondition=initial_condition  SampleTime=Tech
  Q : Outport  InitialOutput=0
  !Q : Outport  Port=2  InitialOutput=1
  wires:
  R/1 -> Mux2/3
  S/1 -> Mux2/2
  Unit Delay1/1 -> Mux2/1
  Demux2/1 -> Unit Delay1/1, Q/1
  Demux2/2 -> !Q/1
  Logic/1 -> Demux2/1
  Mux2/1 -> Logic/1

== system qss_tb_library_aalto/Controller/Gen-set Controller/Engine start control/tempo/S-R Flip-Flop ==
  S : Inport
  R : Inport  Port=2
  Demux2 : Demux  Outputs=2
  Logic : CombinatorialLogic  TruthTable=[0 1;1 0;0 1;0 1;1 0;1 0;0 0;0 0]
  Mux2 : Mux  Inputs=3
  Unit Delay : UnitDelay  InitialCondition=initial_condition  SampleTime=-1
  Q : Outport  InitialOutput=0
  !Q : Outport  Port=2  InitialOutput=1
  wires:
  R/1 -> Mux2/2
  S/1 -> Mux2/1
  Demux2/1 -> Unit Delay/1, Q/1
  Demux2/2 -> !Q/1
  Logic/1 -> Demux2/1
  Mux2/1 -> Logic/1
  Unit Delay/1 -> Mux2/3

== system qss_tb_library_aalto/Controller/Gen-set Controller/Engine start control/tempo/tempo ok --> 1 ==
  S : Inport
  R : Inport  Port=2
  Demux2 : Demux  Outputs=2
  Logic : CombinatorialLogic  TruthTable=[0 1;0 1;1 0;0 1;1 0;0 1;1 0;1 0]
  Mux2 : Mux  Inputs=3
  Unit Delay1 : UnitDelay  InitialCondition=initial_condition  SampleTime=Tech
  Q : Outport  InitialOutput=0
  !Q : Outport  Port=2  InitialOutput=1
  wires:
  Mux2/1 -> Logic/1
  Logic/1 -> Demux2/1
  Demux2/2 -> !Q/1
  Demux2/1 -> Q/1, Unit Delay1/1
  Unit Delay1/1 -> Mux2/1
  S/1 -> Mux2/2
  R/1 -> Mux2/3
